simulink model "Lab_6_LIN_SOLVER"  (R2021a)
settings: Solver=VariableStepAuto  StartTime=0.0  StopTime=double(sim_length)  RelTol=1e-3
undefined symbols (not defined in the file or in its folder): AXI4, Lite
libraries: hdlBasic x60, xbsIndex_r4 x1
settings Model: Creator=ckk5  LastModifiedBy=ckk5

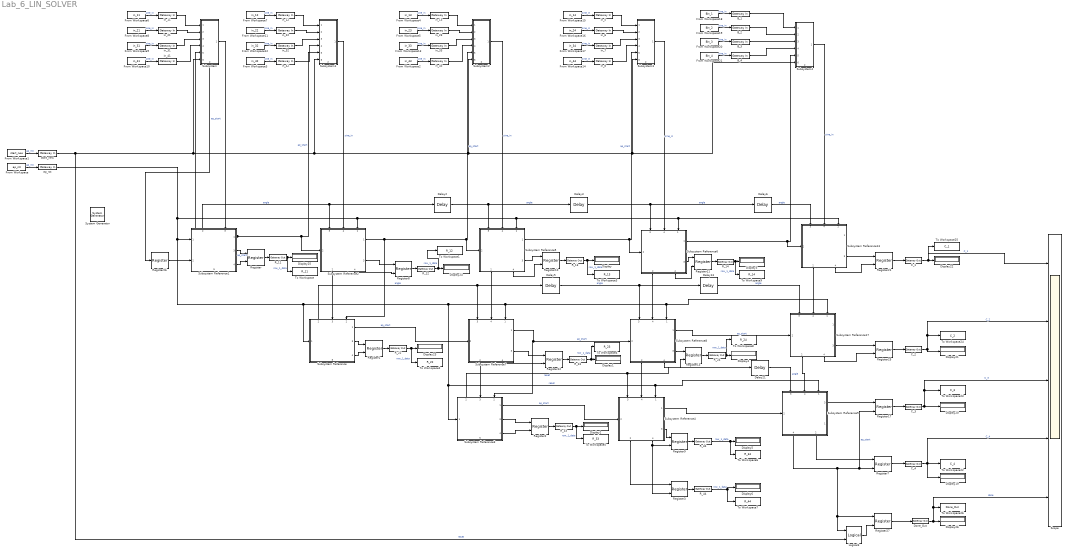
== system Lab_6_LIN_SOLVER ==
  " System Generator" : xbsIndex_r4/ System Generator  Tag=genX  xilinxfamily=zynq  part=xc7z020  speed=-1  package=clg484  synthesis_tool=Vivado  clock_wrapper=Clock Enables  directory=./netlist  proj_type=Vivado  Synth_file=Vivado Synthesis Defaults  Impl_file=Vivado Implementation Defaults  testbench=off  simulink_period=1  sysclk_period=10  dcm_input_clock_period=10  incr_netlist=off  trim_vbits=Everywhere in SubSystem  dbl_ovrd=According to Block Masks  core_generation=According to Block Masks  run_coregen=off  deprecated_control=off  eval_field=0  block_type=sysgen
  B_{1..4} (4 alike) : hdlBasic/Gateway In  gui_display_data_type=Fixed-point  arith_type=Signed (2's comp)  n_bits=16  bin_pt=12  preci_type=Single  exp_width=8  frac_width=24  rows=1  columns=1  quantization="Round  (unbiased: +/- Inf)"  overflow=Saturate  period=1  UseAsADC=off  ADCChannel='1'  interface=AXI4-Lite  automatic_assignment=on  address_offset=hex2dec('00')  intf_name='array_input'  intf_description=''  default_value=0  timing_constraint=None  locs_specified=off  LOCs={}  io_standard={}  inherit_from_input=off  hdl_port=on  XmcBlockStatus=1  maskContainerNames=group4  block_type=gatewayin  block_config=sysgen:gateway_in_config  block_width_w=590  block_height_w=620  block_width=640  block_height=850
  C_{1..4} (4 alike) : hdlBasic/Gateway Out  inherit_from_input=off  hdl_port=on  rows=1  columns=1  UseAsDAC=off  DACChannel='1'  interface=AXI4-Lite  automatic_assignment=on  address_offset=hex2dec('00')  intf_name='output'  intf_description=''  timing_constraint=None  locs_specified=off  LOCs={}  io_standard={}  XmcBlockStatus=1  maskContainerNames=group4  block_type=gatewayout  block_config=sysgen:gateway_out_config  block_width_w=590  block_height_w=620  block_width=620  block_height=750
  Delay{2..3,5..6,13,21} (6 alike) : hdlBasic/Delay  rst=off  en=off  latency=unit_L  reg_retiming=off  XmcBlockStatus=1  maskContainerNames=group1  block_type=delay  block_config=sysgen:Delay_config
  Display{,1..6,19..26} (15 alike) : Display
  Done_Out : hdlBasic/Gateway Out  inherit_from_input=off  hdl_port=on  rows=1  columns=1  UseAsDAC=off  DACChannel='1'  interface=AXI4-Lite  automatic_assignment=on  address_offset=hex2dec('00')  intf_name='control'  intf_description=''  timing_constraint=None  locs_specified=off  LOCs={}  io_standard={}  XmcBlockStatus=1  maskContainerNames=group4  block_type=gatewayout  block_config=sysgen:gateway_out_config  block_width_w=590  block_height_w=620  block_width=620  block_height=750
  From Workspace : FromWorkspace  VariableName=ap_rst  OutputAfterFinalValue=Setting to zero
  From Workspace1 : FromWorkspace  VariableName=start_new  OutputAfterFinalValue=Setting to zero
  From Workspace10 : FromWorkspace  VariableName=in_41  OutputAfterFinalValue=Setting to zero
  From Workspace11 : FromWorkspace  VariableName=in_22  OutputAfterFinalValue=Setting to zero
  From Workspace12 : FromWorkspace  VariableName=in_32  OutputAfterFinalValue=Setting to zero
  From Workspace13 : FromWorkspace  VariableName=in_33  OutputAfterFinalValue=Setting to zero
  From Workspace14 : FromWorkspace  VariableName=in_44  OutputAfterFinalValue=Setting to zero
  From Workspace15 : FromWorkspace  VariableName=in_14  OutputAfterFinalValue=Setting to zero
  From Workspace16 : FromWorkspace  VariableName=in_24  OutputAfterFinalValue=Setting to zero
  From Workspace17 : FromWorkspace  VariableName=in_34  OutputAfterFinalValue=Setting to zero
  From Workspace18 : FromWorkspace  VariableName=Bin_1  OutputAfterFinalValue=Setting to zero
  From Workspace19 : FromWorkspace  VariableName=Bin_2  OutputAfterFinalValue=Setting to zero
  From Workspace2 : FromWorkspace  VariableName=in_43  OutputAfterFinalValue=Setting to zero
  From Workspace20 : FromWorkspace  VariableName=Bin_3  OutputAfterFinalValue=Setting to zero
  From Workspace21 : FromWorkspace  VariableName=Bin_4  OutputAfterFinalValue=Setting to zero
  From Workspace3 : FromWorkspace  VariableName=in_42  OutputAfterFinalValue=Setting to zero
  From Workspace4 : FromWorkspace  VariableName=in_13  OutputAfterFinalValue=Setting to zero
  From Workspace5 : FromWorkspace  VariableName=in_23  OutputAfterFinalValue=Setting to zero
  From Workspace6 : FromWorkspace  VariableName=in_11  OutputAfterFinalValue=Setting to zero
  From Workspace7 : FromWorkspace  VariableName=in_12  OutputAfterFinalValue=Setting to zero
  From Workspace8 : FromWorkspace  VariableName=in_21  OutputAfterFinalValue=Setting to zero
  From Workspace9 : FromWorkspace  VariableName=in_31  OutputAfterFinalValue=Setting to zero
  Logical3 : hdlBasic/Logical  logical_function=OR  inputs=2  en=off  latency=0  precision=Full  arith_type=Unsigned  n_bits=16  bin_pt=0  align_bp=on  overflow=[]  quantization=[]  XmcBlockStatus=1  maskContainerNames=tabcontainer1  block_type=logical  block_config=sysgen:Logical_config
  R_{11..14,22..24,33..34,44} (10 alike) : hdlBasic/Gateway Out  inherit_from_input=off  hdl_port=on  rows=1  columns=1  UseAsDAC=off  DACChannel='1'  interface=AXI4-Lite  automatic_assignment=on  address_offset=hex2dec('00')  intf_name='output'  intf_description=''  timing_constraint=None  locs_specified=off  LOCs={}  io_standard={}  XmcBlockStatus=1  maskContainerNames=group4  block_type=gatewayout  block_config=sysgen:gateway_out_config  block_width_w=590  block_height_w=620  block_width=620  block_height=750
  Register{,1..3,7..13,17,21,25,27} (15 alike) : hdlBasic/Register  init=0  rst=off  en=on  XmcBlockStatus=1  maskContainerNames=tabcontainer1  block_type=register  block_config=sysgen:Register_config
  Register26 : hdlBasic/Register  init=0  rst=off  en=off  XmcBlockStatus=1  maskContainerNames=tabcontainer1  block_type=register  block_config=sysgen:Register_config
  Scope : Scope  NumInputPorts=5
  Subsystem{,1..4} (5 alike) : Subsystem  ReferencedSubsystem=input_muxer
      Subsystem settings: PortSchema="{\"entries\":[{\"content\":{\"sides\":[{\"content\":{\"connectorIds\":[\"In1\",\"In2\",\"In3\",\"In4\",\"In5\",\"In6\"]},\"type\":\"ConnectorPlacement.EquallySpacedRectSide\",\"uuid\":\"c9659870-197e-4708-9e56-aa8d60ec2132\"},{\"content\":{\"connectorIds\":[\"Out1\"],\"side\":\"RIGHT\"},\"type\":\"ConnectorPlacement.EquallySpacedRectSide\",\"uuid\":\"f9d7c189-098f-4a24-828d-c7ef82e0ce16\"},{\"content\":{\"connectorIds\":[],\"side\":\"TOP\"},\"type\":\"ConnectorPlacement.EquallySpacedRectSide\",\"uuid\":\"5053940a-c387-4687-a81e-c4b094664b8d\"},{\"content\":{\"connectorIds\":[\"Out2\"],\"side\":\"BOTTOM\"},\"type\":\"ConnectorPlacement.EquallySpacedRectSide\",\"uuid\":\"4f75bbb3-aea6-4cac-bddf-f1fd262beda3\"}]},\"type\":\"ConnectorPlacement.EquallySpacedConnector\",\"uuid\":\"5b5beda6-ba80-4093-9766-00cb89766bfd\"}],\"packageUris\":[\"http://schema.mathworks.com/mf0/Connector/R2020b\"],\"version\":\"1.0\"}"
      Subsystem1 settings: PortSchema="{\"entries\":[{\"content\":{\"sides\":[{\"content\":{\"connectorIds\":[\"In1\",\"In2\",\"In3\",\"In4\",\"In5\",\"In6\"]},\"type\":\"ConnectorPlacement.EquallySpacedRectSide\",\"uuid\":\"c9659870-197e-4708-9e56-aa8d60ec2132\"},{\"content\":{\"connectorIds\":[\"Out1\"],\"side\":\"RIGHT\"},\"type\":\"ConnectorPlacement.EquallySpacedRectSide\",\"uuid\":\"f9d7c189-098f-4a24-828d-c7ef82e0ce16\"},{\"content\":{\"connectorIds\":[],\"side\":\"TOP\"},\"type\":\"ConnectorPlacement.EquallySpacedRectSide\",\"uuid\":\"5053940a-c387-4687-a81e-c4b094664b8d\"},{\"content\":{\"connectorIds\":[\"Out2\"],\"side\":\"BOTTOM\"},\"type\":\"ConnectorPlacement.EquallySpacedRectSide\",\"uuid\":\"0386b525-0d84-489d-b1ba-c0f65ef89545\"}]},\"type\":\"ConnectorPlacement.EquallySpacedConnector\",\"uuid\":\"5b5beda6-ba80-4093-9766-00cb89766bfd\"}],\"packageUris\":[\"http://schema.mathworks.com/mf0/Connector/R2020b\"],\"version\":\"1.0\"}"
      Subsystem2 settings: PortSchema="{\"entries\":[{\"content\":{\"sides\":[{\"content\":{\"connectorIds\":[\"In1\",\"In2\",\"In3\",\"In4\",\"In5\",\"In6\"]},\"type\":\"ConnectorPlacement.EquallySpacedRectSide\",\"uuid\":\"c9659870-197e-4708-9e56-aa8d60ec2132\"},{\"content\":{\"connectorIds\":[\"Out1\"],\"side\":\"RIGHT\"},\"type\":\"ConnectorPlacement.EquallySpacedRectSide\",\"uuid\":\"f9d7c189-098f-4a24-828d-c7ef82e0ce16\"},{\"content\":{\"connectorIds\":[],\"side\":\"TOP\"},\"type\":\"ConnectorPlacement.EquallySpacedRectSide\",\"uuid\":\"5053940a-c387-4687-a81e-c4b094664b8d\"},{\"content\":{\"connectorIds\":[\"Out2\"],\"side\":\"BOTTOM\"},\"type\":\"ConnectorPlacement.EquallySpacedRectSide\",\"uuid\":\"0b7a346d-dc43-4519-a9aa-7889b337343a\"}]},\"type\":\"ConnectorPlacement.EquallySpacedConnector\",\"uuid\":\"5b5beda6-ba80-4093-9766-00cb89766bfd\"}],\"packageUris\":[\"http://schema.mathworks.com/mf0/Connector/R2020b\"],\"version\":\"1.0\"}"
      Subsystem3 settings: PortSchema="{\"entries\":[{\"content\":{\"sides\":[{\"content\":{\"connectorIds\":[\"In1\",\"In2\",\"In3\",\"In4\",\"In5\",\"In6\"]},\"type\":\"ConnectorPlacement.EquallySpacedRectSide\",\"uuid\":\"c9659870-197e-4708-9e56-aa8d60ec2132\"},{\"content\":{\"connectorIds\":[\"Out1\"],\"side\":\"RIGHT\"},\"type\":\"ConnectorPlacement.EquallySpacedRectSide\",\"uuid\":\"f9d7c189-098f-4a24-828d-c7ef82e0ce16\"},{\"content\":{\"connectorIds\":[],\"side\":\"TOP\"},\"type\":\"ConnectorPlacement.EquallySpacedRectSide\",\"uuid\":\"5053940a-c387-4687-a81e-c4b094664b8d\"},{\"content\":{\"connectorIds\":[\"Out2\"],\"side\":\"BOTTOM\"},\"type\":\"ConnectorPlacement.EquallySpacedRectSide\",\"uuid\":\"96ca4152-851a-4b7b-aabe-a144e8b0fd46\"}]},\"type\":\"ConnectorPlacement.EquallySpacedConnector\",\"uuid\":\"5b5beda6-ba80-4093-9766-00cb89766bfd\"}],\"packageUris\":[\"http://schema.mathworks.com/mf0/Connector/R2020b\"],\"version\":\"1.0\"}"
      Subsystem4 settings: PortSchema="{\"entries\":[{\"content\":{\"sides\":[{\"content\":{\"connectorIds\":[\"In1\",\"In2\",\"In3\",\"In4\",\"In5\",\"In6\"]},\"type\":\"ConnectorPlacement.EquallySpacedRectSide\",\"uuid\":\"c9659870-197e-4708-9e56-aa8d60ec2132\"},{\"content\":{\"connectorIds\":[\"Out1\"],\"side\":\"RIGHT\"},\"type\":\"ConnectorPlacement.EquallySpacedRectSide\",\"uuid\":\"f9d7c189-098f-4a24-828d-c7ef82e0ce16\"},{\"content\":{\"connectorIds\":[],\"side\":\"TOP\"},\"type\":\"ConnectorPlacement.EquallySpacedRectSide\",\"uuid\":\"5053940a-c387-4687-a81e-c4b094664b8d\"},{\"content\":{\"connectorIds\":[\"Out2\"],\"side\":\"BOTTOM\"},\"type\":\"ConnectorPlacement.EquallySpacedRectSide\",\"uuid\":\"96ca4152-851a-4b7b-aabe-a144e8b0fd46\"}]},\"type\":\"ConnectorPlacement.EquallySpacedConnector\",\"uuid\":\"5b5beda6-ba80-4093-9766-00cb89766bfd\"}],\"packageUris\":[\"http://schema.mathworks.com/mf0/Connector/R2020b\"],\"version\":\"1.0\"}"
  Subsystem Reference : Subsystem  ReferencedSubsystem=ATAN_static
      settings: PortSchema="{\"entries\":[{\"content\":{\"sides\":[{\"content\":{\"connectorIds\":[\"In1\"]},\"type\":\"ConnectorPlacement.EquallySpacedRectSide\",\"uuid\":\"e73d0d7d-03bc-4d00-801b-b8c760b16be4\"},{\"content\":{\"connectorIds\":[\"Out1\",\"Out3\",\"Out4\"],\"side\":\"RIGHT\"},\"type\":\"ConnectorPlacement.EquallySpacedRectSide\",\"uuid\":\"fb412951-8b1f-47f8-8fed-40e91e78b205\"},{\"content\":{\"connectorIds\":[\"Out2\",\"In3\",\"In2\"],\"side\":\"TOP\"},\"type\":\"ConnectorPlacement.EquallySpacedRectSide\",\"uuid\":\"8225374e-1161-490d-99ec-3bdc7c7ef343\"},{\"content\":{\"connectorIds\":[\"Out5\"],\"side\":\"BOTTOM\"},\"type\":\"ConnectorPlacement.EquallySpacedRectSide\",\"uuid\":\"cef28eec-a681-4ab7-b320-ffc64443d109\"}]},\"type\":\"ConnectorPlacement.EquallySpacedConnector\",\"uuid\":\"16b5b7a4-aca7-4d8e-a872-8aaff24fa59b\"}],\"packageUris\":[\"http://schema.mathworks.com/mf0/Connector/R2020b\"],\"version\":\"1.0\"}"
  Subsystem Reference1 : Subsystem  ReferencedSubsystem=ATAN_static
      settings: PortSchema="{\"entries\":[{\"content\":{\"sides\":[{\"content\":{\"connectorIds\":[\"In1\",\"In2\"]},\"type\":\"ConnectorPlacement.EquallySpacedRectSide\",\"uuid\":\"e73d0d7d-03bc-4d00-801b-b8c760b16be4\"},{\"content\":{\"connectorIds\":[\"Out1\",\"Out3\",\"Out4\"],\"side\":\"RIGHT\"},\"type\":\"ConnectorPlacement.EquallySpacedRectSide\",\"uuid\":\"fb412951-8b1f-47f8-8fed-40e91e78b205\"},{\"content\":{\"connectorIds\":[\"Out2\",\"In3\"],\"side\":\"TOP\"},\"type\":\"ConnectorPlacement.EquallySpacedRectSide\",\"uuid\":\"8225374e-1161-490d-99ec-3bdc7c7ef343\"},{\"content\":{\"connectorIds\":[\"Out5\"],\"side\":\"BOTTOM\"},\"type\":\"ConnectorPlacement.EquallySpacedRectSide\",\"uuid\":\"cef28eec-a681-4ab7-b320-ffc64443d109\"}]},\"type\":\"ConnectorPlacement.EquallySpacedConnector\",\"uuid\":\"16b5b7a4-aca7-4d8e-a872-8aaff24fa59b\"}],\"packageUris\":[\"http://schema.mathworks.com/mf0/Connector/R2020b\"],\"version\":\"1.0\"}"
  Subsystem Reference{2,4..9,13,17} (9 alike) : Subsystem  ReferencedSubsystem=ROT_static
      Subsystem Reference13 settings: PortSchema="{\"entries\":[{\"content\":{\"sides\":[{\"content\":{\"connectorIds\":[\"In2\"]},\"type\":\"ConnectorPlacement.EquallySpacedRectSide\",\"uuid\":\"e73d0d7d-03bc-4d00-801b-b8c760b16be4\"},{\"content\":{\"connectorIds\":[\"Out1\",\"Out3\"],\"side\":\"RIGHT\"},\"type\":\"ConnectorPlacement.EquallySpacedRectSide\",\"uuid\":\"fb412951-8b1f-47f8-8fed-40e91e78b205\"},{\"content\":{\"connectorIds\":[\"In3\",\"In4\",\"In1\"],\"side\":\"TOP\"},\"type\":\"ConnectorPlacement.EquallySpacedRectSide\",\"uuid\":\"8225374e-1161-490d-99ec-3bdc7c7ef343\"},{\"content\":{\"connectorIds\":[\"Out2\",\"Out4\"],\"side\":\"BOTTOM\"},\"type\":\"ConnectorPlacement.EquallySpacedRectSide\",\"uuid\":\"cef28eec-a681-4ab7-b320-ffc64443d109\"}]},\"type\":\"ConnectorPlacement.EquallySpacedConnector\",\"uuid\":\"16b5b7a4-aca7-4d8e-a872-8aaff24fa59b\"}],\"packageUris\":[\"http://schema.mathworks.com/mf0/Connector/R2020b\"],\"version\":\"1.0\"}"
      Subsystem Reference17 settings: PortSchema="{\"entries\":[{\"content\":{\"sides\":[{\"content\":{\"connectorIds\":[\"In2\"]},\"type\":\"ConnectorPlacement.EquallySpacedRectSide\",\"uuid\":\"e73d0d7d-03bc-4d00-801b-b8c760b16be4\"},{\"content\":{\"connectorIds\":[\"Out1\",\"Out3\"],\"side\":\"RIGHT\"},\"type\":\"ConnectorPlacement.EquallySpacedRectSide\",\"uuid\":\"fb412951-8b1f-47f8-8fed-40e91e78b205\"},{\"content\":{\"connectorIds\":[\"In3\",\"In4\",\"In1\"],\"side\":\"TOP\"},\"type\":\"ConnectorPlacement.EquallySpacedRectSide\",\"uuid\":\"8225374e-1161-490d-99ec-3bdc7c7ef343\"},{\"content\":{\"connectorIds\":[\"Out2\",\"Out4\"],\"side\":\"BOTTOM\"},\"type\":\"ConnectorPlacement.EquallySpacedRectSide\",\"uuid\":\"cef28eec-a681-4ab7-b320-ffc64443d109\"}]},\"type\":\"ConnectorPlacement.EquallySpacedConnector\",\"uuid\":\"16b5b7a4-aca7-4d8e-a872-8aaff24fa59b\"}],\"packageUris\":[\"http://schema.mathworks.com/mf0/Connector/R2020b\"],\"version\":\"1.0\"}"
      Subsystem Reference2 settings: PortSchema="{\"entries\":[{\"content\":{\"sides\":[{\"content\":{\"connectorIds\":[\"In2\"]},\"type\":\"ConnectorPlacement.EquallySpacedRectSide\",\"uuid\":\"e73d0d7d-03bc-4d00-801b-b8c760b16be4\"},{\"content\":{\"connectorIds\":[\"Out1\",\"Out3\"],\"side\":\"RIGHT\"},\"type\":\"ConnectorPlacement.EquallySpacedRectSide\",\"uuid\":\"fb412951-8b1f-47f8-8fed-40e91e78b205\"},{\"content\":{\"connectorIds\":[\"In3\",\"In4\",\"In1\"],\"side\":\"TOP\"},\"type\":\"ConnectorPlacement.EquallySpacedRectSide\",\"uuid\":\"8225374e-1161-490d-99ec-3bdc7c7ef343\"},{\"content\":{\"connectorIds\":[\"Out2\",\"Out4\"],\"side\":\"BOTTOM\"},\"type\":\"ConnectorPlacement.EquallySpacedRectSide\",\"uuid\":\"cef28eec-a681-4ab7-b320-ffc64443d109\"}]},\"type\":\"ConnectorPlacement.EquallySpacedConnector\",\"uuid\":\"16b5b7a4-aca7-4d8e-a872-8aaff24fa59b\"}],\"packageUris\":[\"http://schema.mathworks.com/mf0/Connector/R2020b\"],\"version\":\"1.0\"}"
      Subsystem Reference4 settings: PortSchema="{\"entries\":[{\"content\":{\"sides\":[{\"content\":{\"connectorIds\":[\"In2\"]},\"type\":\"ConnectorPlacement.EquallySpacedRectSide\",\"uuid\":\"e73d0d7d-03bc-4d00-801b-b8c760b16be4\"},{\"content\":{\"connectorIds\":[\"Out1\",\"Out3\"],\"side\":\"RIGHT\"},\"type\":\"ConnectorPlacement.EquallySpacedRectSide\",\"uuid\":\"fb412951-8b1f-47f8-8fed-40e91e78b205\"},{\"content\":{\"connectorIds\":[\"In3\",\"In4\",\"In1\"],\"side\":\"TOP\"},\"type\":\"ConnectorPlacement.EquallySpacedRectSide\",\"uuid\":\"8225374e-1161-490d-99ec-3bdc7c7ef343\"},{\"content\":{\"connectorIds\":[\"Out2\",\"Out4\"],\"side\":\"BOTTOM\"},\"type\":\"ConnectorPlacement.EquallySpacedRectSide\",\"uuid\":\"cef28eec-a681-4ab7-b320-ffc64443d109\"}]},\"type\":\"ConnectorPlacement.EquallySpacedConnector\",\"uuid\":\"16b5b7a4-aca7-4d8e-a872-8aaff24fa59b\"}],\"packageUris\":[\"http://schema.mathworks.com/mf0/Connector/R2020b\"],\"version\":\"1.0\"}"
      Subsystem Reference5 settings: PortSchema="{\"entries\":[{\"content\":{\"sides\":[{\"content\":{\"connectorIds\":[\"In2\"]},\"type\":\"ConnectorPlacement.EquallySpacedRectSide\",\"uuid\":\"e73d0d7d-03bc-4d00-801b-b8c760b16be4\"},{\"content\":{\"connectorIds\":[\"Out1\",\"Out3\"],\"side\":\"RIGHT\"},\"type\":\"ConnectorPlacement.EquallySpacedRectSide\",\"uuid\":\"fb412951-8b1f-47f8-8fed-40e91e78b205\"},{\"content\":{\"connectorIds\":[\"In3\",\"In4\",\"In1\"],\"side\":\"TOP\"},\"type\":\"ConnectorPlacement.EquallySpacedRectSide\",\"uuid\":\"8225374e-1161-490d-99ec-3bdc7c7ef343\"},{\"content\":{\"connectorIds\":[\"Out2\",\"Out4\"],\"side\":\"BOTTOM\"},\"type\":\"ConnectorPlacement.EquallySpacedRectSide\",\"uuid\":\"cef28eec-a681-4ab7-b320-ffc64443d109\"}]},\"type\":\"ConnectorPlacement.EquallySpacedConnector\",\"uuid\":\"16b5b7a4-aca7-4d8e-a872-8aaff24fa59b\"}],\"packageUris\":[\"http://schema.mathworks.com/mf0/Connector/R2020b\"],\"version\":\"1.0\"}"
      Subsystem Reference6 settings: PortSchema="{\"entries\":[{\"content\":{\"sides\":[{\"content\":{\"connectorIds\":[\"In2\"]},\"type\":\"ConnectorPlacement.EquallySpacedRectSide\",\"uuid\":\"e73d0d7d-03bc-4d00-801b-b8c760b16be4\"},{\"content\":{\"connectorIds\":[\"Out1\",\"Out3\"],\"side\":\"RIGHT\"},\"type\":\"ConnectorPlacement.EquallySpacedRectSide\",\"uuid\":\"fb412951-8b1f-47f8-8fed-40e91e78b205\"},{\"content\":{\"connectorIds\":[\"In3\",\"In4\",\"In1\"],\"side\":\"TOP\"},\"type\":\"ConnectorPlacement.EquallySpacedRectSide\",\"uuid\":\"8225374e-1161-490d-99ec-3bdc7c7ef343\"},{\"content\":{\"connectorIds\":[\"Out2\",\"Out4\"],\"side\":\"BOTTOM\"},\"type\":\"ConnectorPlacement.EquallySpacedRectSide\",\"uuid\":\"cef28eec-a681-4ab7-b320-ffc64443d109\"}]},\"type\":\"ConnectorPlacement.EquallySpacedConnector\",\"uuid\":\"16b5b7a4-aca7-4d8e-a872-8aaff24fa59b\"}],\"packageUris\":[\"http://schema.mathworks.com/mf0/Connector/R2020b\"],\"version\":\"1.0\"}"
      Subsystem Reference7 settings: PortSchema="{\"entries\":[{\"content\":{\"sides\":[{\"content\":{\"connectorIds\":[\"In2\"]},\"type\":\"ConnectorPlacement.EquallySpacedRectSide\",\"uuid\":\"e73d0d7d-03bc-4d00-801b-b8c760b16be4\"},{\"content\":{\"connectorIds\":[\"Out1\",\"Out3\"],\"side\":\"RIGHT\"},\"type\":\"ConnectorPlacement.EquallySpacedRectSide\",\"uuid\":\"fb412951-8b1f-47f8-8fed-40e91e78b205\"},{\"content\":{\"connectorIds\":[\"In3\",\"In4\",\"In1\"],\"side\":\"TOP\"},\"type\":\"ConnectorPlacement.EquallySpacedRectSide\",\"uuid\":\"8225374e-1161-490d-99ec-3bdc7c7ef343\"},{\"content\":{\"connectorIds\":[\"Out2\",\"Out4\"],\"side\":\"BOTTOM\"},\"type\":\"ConnectorPlacement.EquallySpacedRectSide\",\"uuid\":\"cef28eec-a681-4ab7-b320-ffc64443d109\"}]},\"type\":\"ConnectorPlacement.EquallySpacedConnector\",\"uuid\":\"16b5b7a4-aca7-4d8e-a872-8aaff24fa59b\"}],\"packageUris\":[\"http://schema.mathworks.com/mf0/Connector/R2020b\"],\"version\":\"1.0\"}"
      Subsystem Reference8 settings: PortSchema="{\"entries\":[{\"content\":{\"sides\":[{\"content\":{\"connectorIds\":[\"In2\"]},\"type\":\"ConnectorPlacement.EquallySpacedRectSide\",\"uuid\":\"e73d0d7d-03bc-4d00-801b-b8c760b16be4\"},{\"content\":{\"connectorIds\":[\"Out1\",\"Out3\"],\"side\":\"RIGHT\"},\"type\":\"ConnectorPlacement.EquallySpacedRectSide\",\"uuid\":\"fb412951-8b1f-47f8-8fed-40e91e78b205\"},{\"content\":{\"connectorIds\":[\"In3\",\"In4\",\"In1\"],\"side\":\"TOP\"},\"type\":\"ConnectorPlacement.EquallySpacedRectSide\",\"uuid\":\"8225374e-1161-490d-99ec-3bdc7c7ef343\"},{\"content\":{\"connectorIds\":[\"Out2\",\"Out4\"],\"side\":\"BOTTOM\"},\"type\":\"ConnectorPlacement.EquallySpacedRectSide\",\"uuid\":\"cef28eec-a681-4ab7-b320-ffc64443d109\"}]},\"type\":\"ConnectorPlacement.EquallySpacedConnector\",\"uuid\":\"16b5b7a4-aca7-4d8e-a872-8aaff24fa59b\"}],\"packageUris\":[\"http://schema.mathworks.com/mf0/Connector/R2020b\"],\"version\":\"1.0\"}"
      Subsystem Reference9 settings: PortSchema="{\"entries\":[{\"content\":{\"sides\":[{\"content\":{\"connectorIds\":[\"In2\"]},\"type\":\"ConnectorPlacement.EquallySpacedRectSide\",\"uuid\":\"e73d0d7d-03bc-4d00-801b-b8c760b16be4\"},{\"content\":{\"connectorIds\":[\"Out3\",\"Out1\"],\"side\":\"RIGHT\"},\"type\":\"ConnectorPlacement.EquallySpacedRectSide\",\"uuid\":\"fb412951-8b1f-47f8-8fed-40e91e78b205\"},{\"content\":{\"connectorIds\":[\"In3\",\"In4\",\"In1\"],\"side\":\"TOP\"},\"type\":\"ConnectorPlacement.EquallySpacedRectSide\",\"uuid\":\"8225374e-1161-490d-99ec-3bdc7c7ef343\"},{\"content\":{\"connectorIds\":[\"Out4\",\"Out2\"],\"side\":\"BOTTOM\"},\"type\":\"ConnectorPlacement.EquallySpacedRectSide\",\"uuid\":\"cef28eec-a681-4ab7-b320-ffc64443d109\"}]},\"type\":\"ConnectorPlacement.EquallySpacedConnector\",\"uuid\":\"16b5b7a4-aca7-4d8e-a872-8aaff24fa59b\"}],\"packageUris\":[\"http://schema.mathworks.com/mf0/Connector/R2020b\"],\"version\":\"1.0\"}"
  Subsystem Reference3 : Subsystem  ReferencedSubsystem=ATAN_static
      settings: PortSchema="{\"entries\":[{\"content\":{\"sides\":[{\"content\":{\"connectorIds\":[\"In1\"]},\"type\":\"ConnectorPlacement.EquallySpacedRectSide\",\"uuid\":\"e73d0d7d-03bc-4d00-801b-b8c760b16be4\"},{\"content\":{\"connectorIds\":[\"Out1\",\"Out3\",\"Out4\"],\"side\":\"RIGHT\"},\"type\":\"ConnectorPlacement.EquallySpacedRectSide\",\"uuid\":\"fb412951-8b1f-47f8-8fed-40e91e78b205\"},{\"content\":{\"connectorIds\":[\"Out2\",\"In3\",\"In2\"],\"side\":\"TOP\"},\"type\":\"ConnectorPlacement.EquallySpacedRectSide\",\"uuid\":\"8225374e-1161-490d-99ec-3bdc7c7ef343\"},{\"content\":{\"connectorIds\":[\"Out5\"],\"side\":\"BOTTOM\"},\"type\":\"ConnectorPlacement.EquallySpacedRectSide\",\"uuid\":\"cef28eec-a681-4ab7-b320-ffc64443d109\"}]},\"type\":\"ConnectorPlacement.EquallySpacedConnector\",\"uuid\":\"16b5b7a4-aca7-4d8e-a872-8aaff24fa59b\"}],\"packageUris\":[\"http://schema.mathworks.com/mf0/Connector/R2020b\"],\"version\":\"1.0\"}"
  To Workspace : ToWorkspace  VariableName=R_11  SaveFormat=Timeseries  SampleTime=-1
  To Workspace1 : ToWorkspace  VariableName=R_12  SaveFormat=Timeseries  SampleTime=-1
  To Workspace2 : ToWorkspace  VariableName=R_22  SaveFormat=Timeseries  SampleTime=-1
  To Workspace22 : ToWorkspace  VariableName=C_4  SaveFormat=Timeseries  SampleTime=-1
  To Workspace23 : ToWorkspace  VariableName=C_3  SaveFormat=Timeseries  SampleTime=-1
  To Workspace24 : ToWorkspace  VariableName=C_2  SaveFormat=Timeseries  SampleTime=-1
  To Workspace25 : ToWorkspace  VariableName=C_1  SaveFormat=Timeseries  SampleTime=-1
  To Workspace26 : ToWorkspace  VariableName=Done_Out  SaveFormat=Timeseries  SampleTime=-1
  To Workspace3 : ToWorkspace  VariableName=R_13  SaveFormat=Timeseries  SampleTime=-1
  To Workspace4 : ToWorkspace  VariableName=R_23  SaveFormat=Timeseries  SampleTime=-1
  To Workspace5 : ToWorkspace  VariableName=R_33  SaveFormat=Timeseries  SampleTime=-1
  To Workspace6 : ToWorkspace  VariableName=R_34  SaveFormat=Timeseries  SampleTime=-1
  To Workspace7 : ToWorkspace  VariableName=R_44  SaveFormat=Timeseries  SampleTime=-1
  To Workspace8 : ToWorkspace  VariableName=R_24  SaveFormat=Timeseries  SampleTime=-1
  To Workspace9 : ToWorkspace  VariableName=R_14  SaveFormat=Timeseries  SampleTime=-1
  ap_rst : hdlBasic/Gateway In  gui_display_data_type=Boolean  arith_type=Boolean  n_bits=16  bin_pt=14  preci_type=Single  exp_width=8  frac_width=24  rows=1  columns=1  quantization="Round  (unbiased: +/- Inf)"  overflow=Saturate  period=1  UseAsADC=off  ADCChannel='1'  interface=AXI4-Lite  automatic_assignment=on  address_offset=hex2dec('00')  intf_name='control'  intf_description=''  default_value=0  timing_constraint=None  locs_specified=off  LOCs={}  io_standard={}  inherit_from_input=off  hdl_port=on  XmcBlockStatus=1  maskContainerNames=group4  block_type=gatewayin  block_config=sysgen:gateway_in_config  block_width_w=590  block_height_w=620  block_width=640  block_height=850
  in_{5..8,11..13,21..23,31..33,41..43} (16 alike) : hdlBasic/Gateway In  gui_display_data_type=Fixed-point  arith_type=Signed (2's comp)  n_bits=16  bin_pt=12  preci_type=Single  exp_width=8  frac_width=24  rows=1  columns=1  quantization="Round  (unbiased: +/- Inf)"  overflow=Saturate  period=1  UseAsADC=off  ADCChannel='1'  interface=AXI4-Lite  automatic_assignment=on  address_offset=hex2dec('00')  intf_name='array_input'  intf_description=''  default_value=0  timing_constraint=None  locs_specified=off  LOCs={}  io_standard={}  inherit_from_input=off  hdl_port=on  XmcBlockStatus=1  maskContainerNames=group4  block_type=gatewayin  block_config=sysgen:gateway_in_config  block_width_w=590  block_height_w=620  block_width=640  block_height=850
  start_new : hdlBasic/Gateway In  gui_display_data_type=Boolean  arith_type=Boolean  n_bits=16  bin_pt=14  preci_type=Single  exp_width=8  frac_width=24  rows=1  columns=1  quantization="Round  (unbiased: +/- Inf)"  overflow=Saturate  period=1  UseAsADC=off  ADCChannel='1'  interface=AXI4-Lite  automatic_assignment=on  address_offset=hex2dec('00')  intf_name='control'  intf_description=''  default_value=0  timing_constraint=None  locs_specified=off  LOCs={}  io_standard={}  inherit_from_input=off  hdl_port=on  XmcBlockStatus=1  maskContainerNames=group4  block_type=gatewayin  block_config=sysgen:gateway_in_config  block_width_w=590  block_height_w=620  block_width=640  block_height=850
  wires:
  From Workspace/1 -> ap_rst/1  "ap_rst"
  Subsystem1/1 -> Subsystem Reference2/4  "sine_in"
  Subsystem Reference2/2 -> Subsystem Reference/3
  Delay2/1 -> Delay3/1, Subsystem Reference5/3  "angle"
  Subsystem2/1 -> Subsystem Reference5/4  "sine_in"
  Subsystem Reference2/1 -> Subsystem Reference5/2, Subsystem2/5, Subsystem Reference/2  "ap_start"
  Subsystem3/1 -> Subsystem Reference6/4  "sine_in"
  Subsystem Reference5/1 -> Subsystem Reference6/2, Subsystem3/5  "ap_start"
  Subsystem Reference/1 -> Subsystem Reference7/2  "ap_start"
  Subsystem Reference/2 -> Delay5/1, Subsystem Reference7/3  "angle"
  Delay5/1 -> Delay13/1, Subsystem Reference8/3  "angle"
  Subsystem Reference7/1 -> Subsystem Reference8/2, Subsystem Reference3/2  "ap_start"
  Subsystem Reference3/1 -> Subsystem Reference4/2  "ap_start"
  Delay6/1 -> Subsystem Reference13/3  "angle"
  Delay3/1 -> Delay6/1, Subsystem Reference6/3  "angle"
  Subsystem Reference6/1 -> Subsystem4/5, Subsystem Reference13/2
  Delay13/1 -> Subsystem Reference17/3  "angle"
  Subsystem Reference8/2 -> Subsystem Reference4/4
  Subsystem Reference7/2 -> Subsystem Reference3/3
  Subsystem Reference6/2 -> Subsystem Reference8/4
  Subsystem Reference5/2 -> Subsystem Reference7/4
  Delay21/1 -> Subsystem Reference9/3  "angle"
  Subsystem Reference3/2 -> Delay21/1, Subsystem Reference4/3  "reset"
  Subsystem Reference4/1 -> Subsystem Reference9/2
  Subsystem Reference17/2 -> Subsystem Reference9/4
  ap_rst/1 -> Subsystem Reference/1, Subsystem Reference3/1, Subsystem Reference4/1, Subsystem Reference9/1, Subsystem Reference17/1, Subsystem Reference8/1, Subsystem Reference7/1, Subsystem Reference1/1, Subsystem Reference2/1, Subsystem Reference13/1, Subsystem Reference6/1, Subsystem Reference5/1  "reset"
  Subsystem Reference4/2 -> Register3/1
  Subsystem Reference4/4 -> Register9/2, Register3/2
  Register/1 -> R_11/1
  Subsystem Reference1/1 -> Subsystem Reference2/2, Subsystem1/5, Subsystem/5  "ap_start"
  Subsystem Reference1/2 -> Subsystem Reference2/3, Delay2/1  "angle"
  Register1/1 -> R_22/1
  Subsystem Reference/4 -> Register1/2
  Subsystem Reference/3 -> Register1/1
  Subsystem Reference3/4 -> Register2/2
  Register2/1 -> R_33/1
  Subsystem Reference3/3 -> Register2/1
  Register3/1 -> R_44/1
  Register7/1 -> C_4/1
  Register8/1 -> R_12/1
  Subsystem Reference2/4 -> Register8/2
  Subsystem Reference2/3 -> Register8/1
  Register9/1 -> R_34/1
  Subsystem Reference4/3 -> Register9/1
  Register10/1 -> R_13/1
  Subsystem Reference5/3 -> Register10/1
  Subsystem Reference5/4 -> Register10/2
  Register11/1 -> R_14/1
  Subsystem Reference6/3 -> Register11/1
  Subsystem Reference6/4 -> Register11/2
  Register12/1 -> R_23/1
  Subsystem Reference7/3 -> Register12/1
  Subsystem Reference7/4 -> Register12/2
  Register13/1 -> R_24/1
  Subsystem Reference8/3 -> Register13/1
  Subsystem Reference8/4 -> Register13/2
  Subsystem Reference9/3 -> Register17/1
  Register17/1 -> C_3/1
  Subsystem Reference13/3 -> Register21/1
  Subsystem Reference13/4 -> Register21/2
  Register21/1 -> C_1/1
  Subsystem Reference17/3 -> Register25/1
  Subsystem Reference17/4 -> Register25/2
  Register25/1 -> C_2/1
  Subsystem Reference13/2 -> Subsystem Reference17/4
  Subsystem Reference8/1 -> Subsystem Reference17/2  "ap_start"
  R_13/1 -> To Workspace3/1, Display/1  "row_1_data"
  R_23/1 -> To Workspace4/1, Display1/1  "row_1_data"
  R_33/1 -> To Workspace5/1, Display2/1  "row_1_data"
  R_14/1 -> To Workspace9/1, Display3/1  "row_1_data"
  R_24/1 -> To Workspace8/1, Display4/1  "row_1_data"
  R_34/1 -> To Workspace6/1, Display5/1  "row_1_data"
  R_44/1 -> Display6/1, To Workspace7/1  "row_1_data"
  C_4/1 -> Display19/1, Scope/4, To Workspace22/1  "C_4"
  C_3/1 -> To Workspace23/1, Scope/3, Display20/1  "C_3"
  C_2/1 -> Scope/2, To Workspace24/1, Display21/1  "C_2"
  C_1/1 -> Scope/1, To Workspace25/1, Display22/1  "C_1"
  R_22/1 -> To Workspace2/1, Display23/1  "row_1_data"
  R_12/1 -> To Workspace1/1, Display24/1  "row_1_data"
  R_11/1 -> To Workspace/1, Display25/1  "row_1_data"
  From Workspace6/1 -> in_11/1  "sine_in"
  From Workspace8/1 -> in_21/1  "sine_in"
  From Workspace9/1 -> in_31/1  "sine_in"
  From Workspace10/1 -> in_41/1  "sine_in"
  in_11/1 -> Subsystem/1
  in_21/1 -> Subsystem/2
  in_31/1 -> Subsystem/3
  in_41/1 -> Subsystem/4
  Subsystem/1 -> Subsystem Reference1/3
  in_32/1 -> Subsystem1/3
  in_22/1 -> Subsystem1/2
  in_42/1 -> Subsystem1/4
  in_12/1 -> Subsystem1/1
  From Workspace7/1 -> in_12/1  "sine_in"
  From Workspace12/1 -> in_32/1  "sine_in"
  From Workspace3/1 -> in_42/1  "sine_in"
  From Workspace11/1 -> in_22/1  "sine_in"
  in_33/1 -> Subsystem2/3
  in_23/1 -> Subsystem2/2
  in_43/1 -> Subsystem2/4
  in_13/1 -> Subsystem2/1
  From Workspace4/1 -> in_13/1  "sine_in"
  From Workspace13/1 -> in_33/1  "sine_in"
  From Workspace2/1 -> in_43/1  "sine_in"
  From Workspace5/1 -> in_23/1  "sine_in"
  in_7/1 -> Subsystem3/3
  in_6/1 -> Subsystem3/2
  in_8/1 -> Subsystem3/4
  in_5/1 -> Subsystem3/1
  From Workspace15/1 -> in_5/1  "sine_in"
  From Workspace17/1 -> in_7/1  "sine_in"
  From Workspace14/1 -> in_8/1  "sine_in"
  From Workspace16/1 -> in_6/1  "sine_in"
  Subsystem/2 -> Register26/1  "ap_start"
  Subsystem Reference1/4 -> Register/2
  Subsystem Reference1/3 -> Register/1  "ap_start"
  Register26/1 -> Subsystem Reference1/2
  B_1/1 -> Subsystem4/1
  B_2/1 -> Subsystem4/2
  B_4/1 -> Subsystem4/4
  B_3/1 -> Subsystem4/3
  Subsystem4/1 -> Subsystem Reference13/4  "sine_in"
  From Workspace1/1 -> start_new/1  "ap_rst"
  start_new/1 -> Logical3/2, Subsystem1/6, Subsystem2/6, Subsystem4/6, Subsystem3/6, Subsystem/6  "reset"
  Register27/1 -> Done_Out/1
  Logical3/1 -> Register27/2
  Done_Out/1 -> Scope/5, To Workspace26/1, Display26/1  "done"
  From Workspace18/1 -> B_1/1  "sine_in"
  Subsystem Reference9/2 -> Register7/1
  Subsystem Reference9/4 -> Logical3/1, Register27/1, Register17/2, Register7/2  "ap_start"
  From Workspace19/1 -> B_2/1  "sine_in"
  From Workspace20/1 -> B_3/1  "sine_in"
  From Workspace21/1 -> B_4/1  "sine_in"
